simulink model "Implausibility_ETR07_Study"  (R2017b)
settings: Solver=FixedStepAuto  StartTime=0.0  StopTime=10.0  RelTol=1e-3
settings Model: Creator=cspt  LastModifiedBy=cspt
settings RTWCC: SystemTargetFile=irt.tlc  TemplateMakefile=irt_default_tmf  Description=INTECRIO Real-Time Target
settings STFCustomTargetCC: TargetLangStandard=C99 (ISO)  UtilityFuncGeneration=Shared location  SystemTargetFile=irt.tlc
settings GRTTargetCC: UtilityFuncGeneration=Shared location  ParMdlRefBuildCompliant=off  CompOptLevelCompliant=off  ConcurrentExecutionCompliant=off  CombineOutputUpdateFcns=off  MatFileLogging=off  CPPClassGenCompliant=off  GRTInterface=on  UseToolchainInfoCompliant=off  GenerateASAP2=on

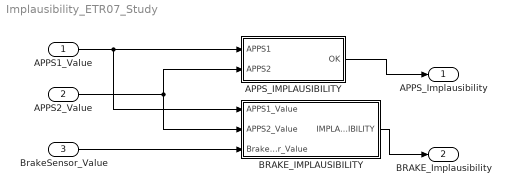
== system Implausibility_ETR07_Study ==
  APPS1_Value : Inport
  APPS2_Value : Inport  Port=2
  BrakeSensor_Value : Inport  Port=3
  APPS_IMPLAUSIBILITY : Subsystem
  BRAKE_IMPLAUSIBILITY : Subsystem
  APPS_Implausibility : Outport
  BRAKE_Implausibility : Outport  Port=2
  wires:
  BRAKE_IMPLAUSIBILITY/1(IMPLAUSIBILITY) -> BRAKE_Implausibility/1
  APPS2_Value/1 -> BRAKE_IMPLAUSIBILITY/2(APPS2_Value), APPS_IMPLAUSIBILITY/2(APPS2)
  APPS1_Value/1 -> BRAKE_IMPLAUSIBILITY/1(APPS1_Value), APPS_IMPLAUSIBILITY/1(APPS1)
  APPS_IMPLAUSIBILITY/1(OK) -> APPS_Implausibility/1
  BrakeSensor_Value/1 -> BRAKE_IMPLAUSIBILITY/3(BrakeSensor_Value)

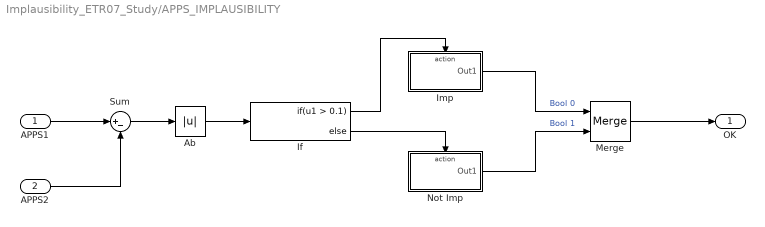
== system Implausibility_ETR07_Study/APPS_IMPLAUSIBILITY ==
  APPS1 : Inport
  APPS2 : Inport  Port=2
  Ab : Abs
  If : If  IfExpression=u1 > 0.1
  Imp : Subsystem  TreatAsAtomicUnit=on
  Merge : Merge
  Not Imp : Subsystem  TreatAsAtomicUnit=on
  Sum : Sum  Inputs=|+-
  OK : Outport
  wires:
  APPS1/1 -> Sum/1
  APPS2/1 -> Sum/2
  Sum/1 -> Ab/1
  Ab/1 -> If/1
  Imp/1(Out1) -> Merge/1  "Bool 0"
  Not Imp/1(Out1) -> Merge/2  "Bool 1"
  Merge/1 -> OK/1
  If/2 -> Not Imp/Action
  If/1 -> Imp/Action

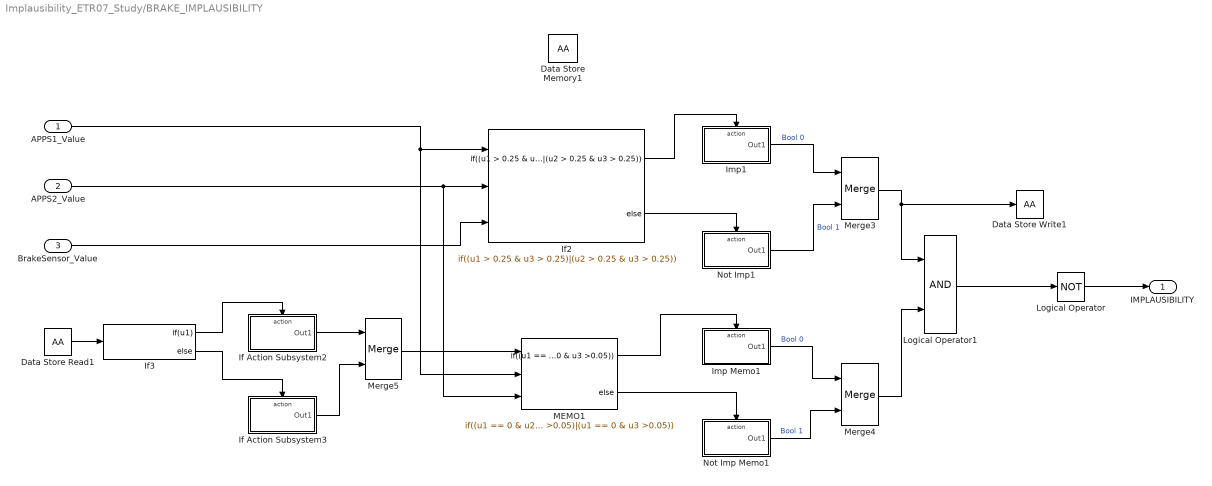
== system Implausibility_ETR07_Study/BRAKE_IMPLAUSIBILITY ==
  APPS1_Value : Inport
  APPS2_Value : Inport  Port=2
  BrakeSensor_Value : Inport  Port=3
  Data Store Memory1 : DataStoreMemory  DataStoreName=AA  ReadBeforeWriteMsg=warning  WriteAfterWriteMsg=warning  WriteAfterReadMsg=warning  ShowAdditionalParam=off
  Data Store Read1 : DataStoreRead  DataStoreName=AA
  Data Store Write1 : DataStoreWrite  DataStoreName=AA
  If Action Subsystem2 : Subsystem  TreatAsAtomicUnit=on
  If Action Subsystem3 : Subsystem  TreatAsAtomicUnit=on
  If2 : If  NumInputs=3  IfExpression=(u1 > 0.25 & u3 > 0.25)|(u2 > 0.25 & u3 > 0.25)
  If3 : If  IfExpression=u1
  Imp Memo1 : Subsystem  TreatAsAtomicUnit=on
  Imp1 : Subsystem  TreatAsAtomicUnit=on
  Logical Operator : Logic  Operator=NOT  IconShape=distinctive  AllPortsSameDT=off  OutDataTypeStr=boolean
  Logical Operator1 : Logic  OutDataTypeStr=boolean
  MEMO1 : If  NumInputs=3  IfExpression=(u1 == 0 & u2 >0.05)|(u1 == 0 & u3 >0.05)
  Merge3 : Merge
  Merge4 : Merge
  Merge5 : Merge
  Not Imp Memo1 : Subsystem  TreatAsAtomicUnit=on
  Not Imp1 : Subsystem  TreatAsAtomicUnit=on
  IMPLAUSIBILITY : Outport
  wires:
  Imp Memo1/1(Out1) -> Merge4/1  "Bool 0"
  Data Store Read1/1 -> If3/1
  Merge5/1 -> MEMO1/1
  If3/1 -> If Action Subsystem2/Action
  If Action Subsystem3/1(Out1) -> Merge5/2
  Imp1/1(Out1) -> Merge3/1  "Bool 0"
  If3/2 -> If Action Subsystem3/Action
  Not Imp Memo1/1(Out1) -> Merge4/2  "Bool 1"
  Not Imp1/1(Out1) -> Merge3/2  "Bool 1"
  If2/2 -> Not Imp1/Action
  If2/1 -> Imp1/Action
  MEMO1/2 -> Not Imp Memo1/Action
  Merge3/1 -> Data Store Write1/1, Logical Operator1/1
  BrakeSensor_Value/1 -> If2/3
  APPS2_Value/1 -> MEMO1/3, If2/2
  MEMO1/1 -> Imp Memo1/Action
  If Action Subsystem2/1(Out1) -> Merge5/1
  Merge4/1 -> Logical Operator1/2
  APPS1_Value/1 -> MEMO1/2, If2/1
  Logical Operator1/1 -> Logical Operator/1
  Logical Operator/1 -> IMPLAUSIBILITY/1

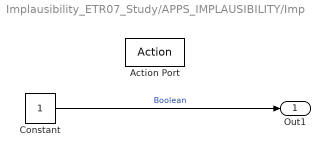
== system Implausibility_ETR07_Study/APPS_IMPLAUSIBILITY/Imp ==
  Action Port : ActionPort  ActionType=then
  Constant : Constant  OutDataTypeStr=boolean
  Out1 : Outport
  wires:
  Constant/1 -> Out1/1  "Boolean"

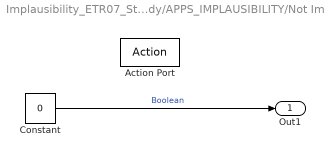
== system Implausibility_ETR07_Study/APPS_IMPLAUSIBILITY/Not Imp ==
  Action Port : ActionPort  ActionType=else
  Constant : Constant  Value=0  OutDataTypeStr=boolean
  Out1 : Outport
  wires:
  Constant/1 -> Out1/1  "Boolean"

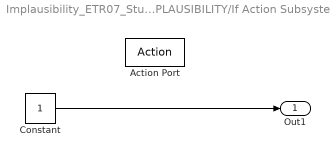
== system Implausibility_ETR07_Study/BRAKE_IMPLAUSIBILITY/If Action Subsystem2 ==
  Action Port : ActionPort  ActionType=then
  Constant : Constant
  Out1 : Outport
  wires:
  Constant/1 -> Out1/1

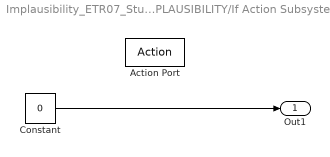
== system Implausibility_ETR07_Study/BRAKE_IMPLAUSIBILITY/If Action Subsystem3 ==
  Action Port : ActionPort  ActionType=else
  Constant : Constant  Value=0
  Out1 : Outport
  wires:
  Constant/1 -> Out1/1

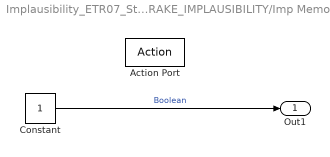
== system Implausibility_ETR07_Study/BRAKE_IMPLAUSIBILITY/Imp Memo1 ==
  Action Port : ActionPort  ActionType=then
  Constant : Constant  OutDataTypeStr=boolean
  Out1 : Outport
  wires:
  Constant/1 -> Out1/1  "Boolean"

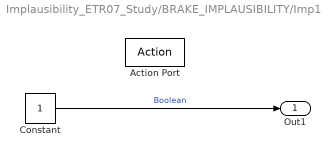
== system Implausibility_ETR07_Study/BRAKE_IMPLAUSIBILITY/Imp1 ==
  Action Port : ActionPort  ActionType=then
  Constant : Constant  OutDataTypeStr=boolean
  Out1 : Outport
  wires:
  Constant/1 -> Out1/1  "Boolean"

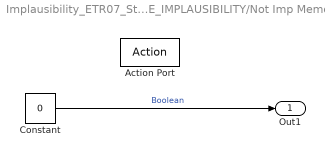
== system Implausibility_ETR07_Study/BRAKE_IMPLAUSIBILITY/Not Imp Memo1 ==
  Action Port : ActionPort  ActionType=else
  Constant : Constant  Value=0  OutDataTypeStr=boolean
  Out1 : Outport
  wires:
  Constant/1 -> Out1/1  "Boolean"

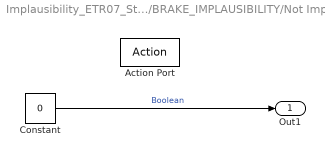
== system Implausibility_ETR07_Study/BRAKE_IMPLAUSIBILITY/Not Imp1 ==
  Action Port : ActionPort  ActionType=else
  Constant : Constant  Value=0  OutDataTypeStr=boolean
  Out1 : Outport
  wires:
  Constant/1 -> Out1/1  "Boolean"
